simulink model "verify_Pressuredrop_mdl"  (R2016b)
settings: Solver=VariableStepDiscrete  StartTime=0.0  StopTime=100  MaxStep=1  RelTol=1e-3  EnableMultiTasking=on
libraries: carnot x1, simulink x1
settings Model: Creator=drhf  LastModifiedBy=drhf
settings DataIOCC: LimitDataPoints=on  SaveFormat=Array  SignalLoggingSaveFormat=ModelDataLogs
settings OptimizationCC: ExpressionDepthLimit=2147483647  LifeSpan=inf
settings DebuggingCC: UnderspecifiedInitializationDetection=Classic  MergeDetectMultiDrivingBlocksExec=none  SolverPrmCheckMsg=warning  FcnCallInpInsideContextMsg=warning  StateNameClashWarn=warning  SFUnexpectedBacktrackingDiag=warning  SFNoUnconditionalDefaultTransitionDiag=warning  SFExecutionAtInitializationDiag=none
settings HardwareCC: ProdBitPerPointer=32  ProdBitPerSizeT=32  ProdBitPerPtrDiffT=32  ProdLargestAtomicFloat=None  ProdIntDivRoundTo=Undefined  ProdEndianess=Unspecified  ProdWordSize=32  ProdHWDeviceType=32-bit Generic
settings ModelReferenceCC: PropagateSignalLabelsOutOfModel=off
settings GRTTargetCC: TargetLangStandard=C89/C90 (ANSI)  GeneratePreprocessorConditionals=Disable all  CombineOutputUpdateFcns=off  GRTInterface=on
settings ConfigComp: CovMetricSettings=dw  CovHtmlReporting=on  CovSaveCumulativeToWorkspaceVar=on  CovSaveSingleToWorkspaceVar=on  CovExternalEMLEnable=off

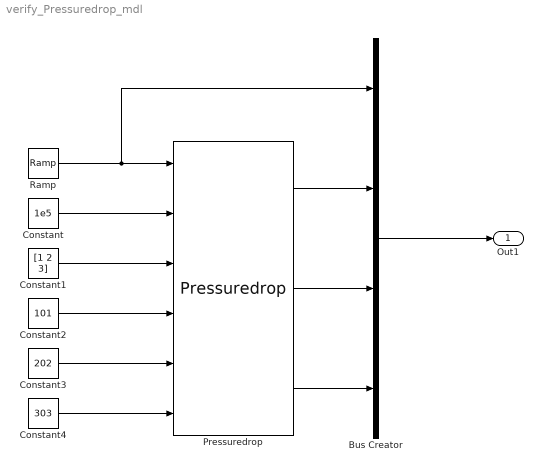
== system verify_Pressuredrop_mdl ==
  Bus Creator : BusCreator  Inputs=4
  Constant : Constant  Value=1e5
  Constant1 : Constant  Value=[1 2 3]
  Constant2 : Constant  Value=101
  Constant3 : Constant  Value=202
  Constant4 : Constant  Value=303
  Pressuredrop : carnot/Basic/Pressure_Drop/Pressuredrop
  Ramp : simulink/Sources/Ramp  slope=0.01  start=0  X0=0
  Out1 : Outport
  wires:
  Bus Creator/1 -> Out1/1
  Pressuredrop/1 -> Bus Creator/2
  Pressuredrop/2 -> Bus Creator/3
  Pressuredrop/3 -> Bus Creator/4
  Constant/1 -> Pressuredrop/2
  Constant1/1 -> Pressuredrop/3
  Constant2/1 -> Pressuredrop/4
  Constant3/1 -> Pressuredrop/5
  Constant4/1 -> Pressuredrop/6
  Ramp/1 -> Bus Creator/1, Pressuredrop/1
